simulink model "projekt1_"  (R2016b)
settings: Solver=VariableStepAuto  StartTime=0.0  StopTime=100  RelTol=1e-3
values from neighbouring files (symbols this model uses):
  Tp = 1    [projekt1.m]    (also in projekt1_5.m)
  u_ = 2    [projekt1.m]    (also in projekt1_5.m = 0)
settings Model: Creator=m  LastModifiedBy=m

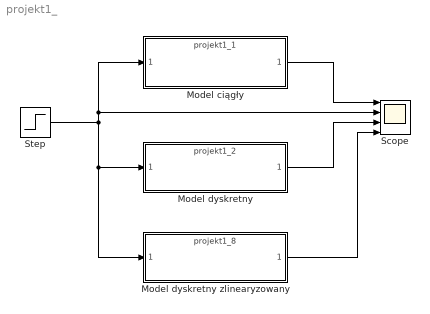
== system projekt1_ ==
  Model ciągły : ModelReference  ModelNameDialog=projekt1_1.slx  SimulationMode=Normal  ModelReferenceVersion=1.11
  Model dyskretny : ModelReference  ModelNameDialog=projekt1_2  SimulationMode=Normal  ModelReferenceVersion=1.6
  Model dyskretny zlinearyzowany : ModelReference  ModelNameDialog=projekt1_8  SimulationMode=Normal  ModelReferenceVersion=1.10
  Scope : Scope  NumInputPorts=4
  Step : Step  After=u_  SampleTime=Tp
  wires:
  Step/1 -> Scope/2, Model ciągły/1, Model dyskretny zlinearyzowany/1, Model dyskretny/1
  Model ciągły/1 -> Scope/1
  Model dyskretny/1 -> Scope/3
  Model dyskretny zlinearyzowany/1 -> Scope/4
